simulink model "simu2"  (R2020b)
settings: Solver=VariableStepAuto  StartTime=0.0  StopTime=Ttt  MaxStep=0.01  RelTol=1e-3
values from neighbouring files (symbols this model uses):
  A = 1    [lab2.m]
libraries: simulink x2
settings Model: Creator=pkubo  LastModifiedBy=pkubo
settings DataIOCC: ReturnWorkspaceOutputs=off

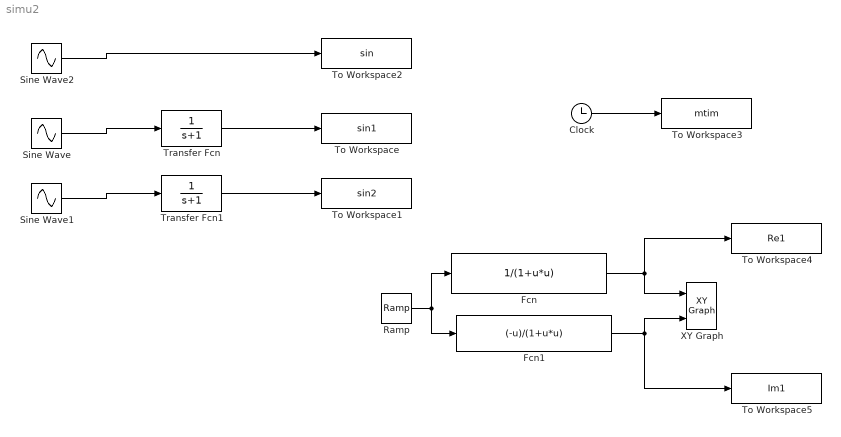
== system simu2 ==
  Clock : Clock
  Fcn : Fcn  Expr=1/(1+u*u)
  Fcn1 : Fcn  Expr=(-u)/(1+u*u)
  Ramp : simulink/Sources/Ramp  slope=1  start=0  InitialOutput=0
  Sine Wave : Sin  SampleTime=0
  Sine Wave1 : Sin  Amplitude=A  Frequency=2  SampleTime=0
  Sine Wave2 : Sin  SampleTime=0
  To Workspace : ToWorkspace  VariableName=sin1  SampleTime=-1
  To Workspace1 : ToWorkspace  VariableName=sin2  SampleTime=-1
  To Workspace2 : ToWorkspace  VariableName=sin  SampleTime=-1
  To Workspace3 : ToWorkspace  VariableName=mtim  SampleTime=-1
  To Workspace4 : ToWorkspace  VariableName=Re1  SampleTime=-1
  To Workspace5 : ToWorkspace  VariableName=Im1  SampleTime=-1
  Transfer Fcn : TransferFcn  Denominator=[1 1]
  Transfer Fcn1 : TransferFcn  Denominator=[1 1]
  XY Graph : simulink/Sinks/XY Graph  xmin=-1  xmax=1  ymin=-1  ymax=1  st=-1
  wires:
  Sine Wave/1 -> Transfer Fcn/1
  Transfer Fcn/1 -> To Workspace/1
  Clock/1 -> To Workspace3/1
  Transfer Fcn1/1 -> To Workspace1/1
  Sine Wave1/1 -> Transfer Fcn1/1
  Sine Wave2/1 -> To Workspace2/1
  Fcn1/1 -> To Workspace5/1, XY Graph/2
  Ramp/1 -> Fcn1/1, Fcn/1
  Fcn/1 -> To Workspace4/1, XY Graph/1
